simulink model "harmonics"  (R2025b)
settings: Solver=ode14x  StartTime=0.0  StopTime=0.2  FixedStep=1e-5  RelTol=1e-3
values from neighbouring files (symbols this model uses):
  f = 50.0    [ctrlSys.sldd]
  Ts_local = 1.0E-5    [ctrlSys.sldd]
libraries: eeRmsMeasurement x2
settings Model: DataDictionary=ctrlSys.sldd  Creator=LYG  LastModifiedBy=i336

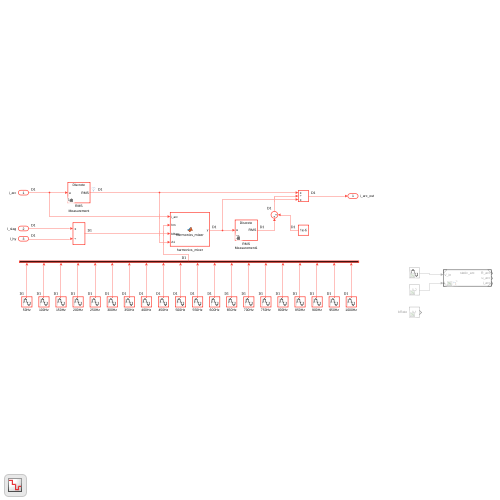
[thumbnail: Simulink's stored preview of the top-level diagram]
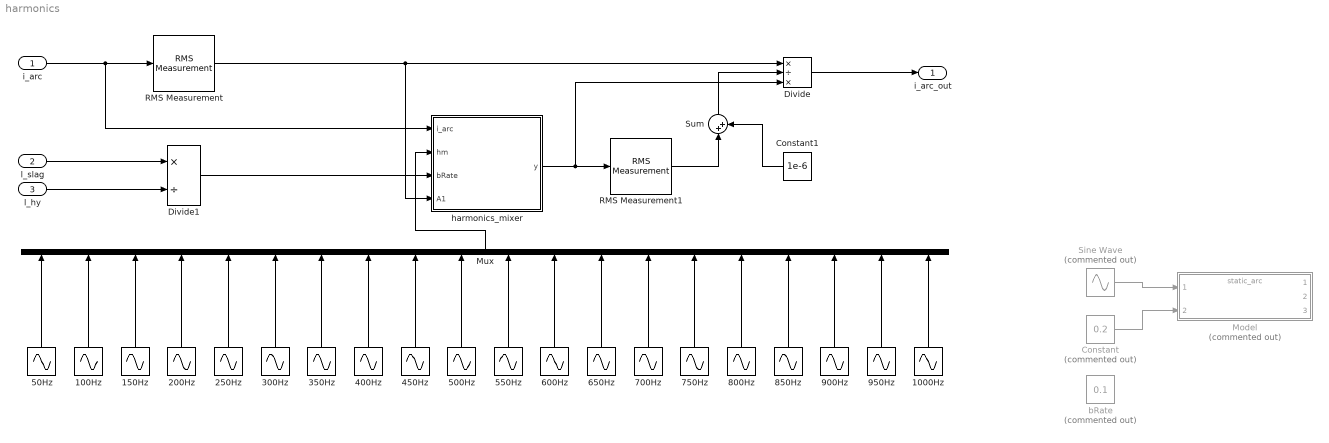
== system harmonics ==
  i_arc : Inport
  l_slag : Inport  Port=2
  l_hy : Inport  Port=3  PortDimensions=3
  1000Hz : Sin  Frequency=2 * pi * f * 20  Phase=-0.6225  SampleTime=Ts_local
  100Hz : Sin  Frequency=2 * pi * f * 2  Phase=-0.4679  SampleTime=Ts_local
  150Hz : Sin  Frequency=2 * pi * f * 3  Phase=-0.8069  SampleTime=Ts_local
  200Hz : Sin  Frequency=2 * pi * f * 4  Phase=0.0685  SampleTime=Ts_local
  250Hz : Sin  Frequency=2 * pi * f * 5  Phase=-1.3175  SampleTime=Ts_local
  300Hz : Sin  Frequency=2 * pi * f * 6  Phase=-0.0827  SampleTime=Ts_local
  350Hz : Sin  Frequency=2 * pi * f * 7  Phase=-1.1120  SampleTime=Ts_local
  400Hz : Sin  Frequency=2 * pi * f * 8  Phase=-0.4285  SampleTime=Ts_local
  450Hz : Sin  Frequency=2 * pi * f * 9  Phase=-1.5794  SampleTime=Ts_local
  500Hz : Sin  Frequency=2 * pi * f * 10  Phase=-0.2913  SampleTime=Ts_local
  50Hz : Sin  Frequency=2 * pi * f * 1  Phase=-2.2678  SampleTime=Ts_local
  550Hz : Sin  Frequency=2 * pi * f * 11  Phase=-1.9727  SampleTime=Ts_local
  600Hz : Sin  Frequency=2 * pi * f * 12  Phase=-0.4659  SampleTime=Ts_local
  650Hz : Sin  Frequency=2 * pi * f * 13  Phase=-2.1009  SampleTime=Ts_local
  700Hz : Sin  Frequency=2 * pi * f * 14  Phase=-0.5103  SampleTime=Ts_local
  750Hz : Sin  Frequency=2 * pi * f * 15  Phase=-2.4781  SampleTime=Ts_local
  800Hz : Sin  Frequency=2 * pi * f * 16  Phase=-0.5504  SampleTime=Ts_local
  850Hz : Sin  Frequency=2 * pi * f * 17  Phase=-2.8439  SampleTime=Ts_local
  900Hz : Sin  Frequency=2 * pi * f * 18  Phase=-0.6115  SampleTime=Ts_local
  950Hz : Sin  Frequency=2 * pi * f * 19  Phase=3.1081  SampleTime=Ts_local
  Constant : Constant  Commented=on  Value=0.2  SampleTime=1e-5
  Constant1 : Constant  Value=1e-6  SampleTime=Ts_local
  Divide : Product  Inputs=*/*
  Divide1 : Product  Inputs=*/
  Model : ModelReference  Commented=on  ModelNameDialog=static_arc.slx  SimulationMode=Normal  ModelReferenceVersion=1.10
  Mux : Mux  Inputs=20
  RMS Measurement : eeRmsMeasurement/RMS Measurement  LabelModeActiveChoice=Total  F=f  SpecifyHarmonics=off  K=[0 1 2]  Ts=Ts_local
      settings: LibrarySourceBlock=|
      | ee_sl_lib/Measurements/RMS
      | Measurement
  RMS Measurement1 : eeRmsMeasurement/RMS Measurement  LabelModeActiveChoice=Total  F=f  SpecifyHarmonics=off  K=[0 1]  Ts=Ts_local
      settings: LibrarySourceBlock=|
      | ee_sl_lib/Measurements/RMS
      | Measurement
  Sine Wave : Sin  Commented=on  Amplitude=sqrt(2) * 650  Frequency=2 * pi * 50  SampleTime=1e-5
  Sum : Sum  Inputs=|++
  bRate : Constant  Commented=on  Value=0.1  SampleTime=1e-5
  harmonics_mixer : MATLAB Function  TreatAsAtomicUnit=on  SystemSampleTime=Ts_local
  i_arc_out : Outport
  wires:
  Sine Wave/1 -> Model/1
  Constant/1 -> Model/2
  50Hz/1 -> Mux/1
  100Hz/1 -> Mux/2
  150Hz/1 -> Mux/3
  200Hz/1 -> Mux/4
  250Hz/1 -> Mux/5
  300Hz/1 -> Mux/6
  350Hz/1 -> Mux/7
  400Hz/1 -> Mux/8
  450Hz/1 -> Mux/9
  500Hz/1 -> Mux/10
  Mux/1 -> harmonics_mixer/2(hm)
  RMS Measurement/1 -> Divide/1, harmonics_mixer/4(A1)
  harmonics_mixer/1(y) -> Divide/3, RMS Measurement1/1
  Sum/1 -> Divide/2
  RMS Measurement1/1 -> Sum/1
  Constant1/1 -> Sum/2
  550Hz/1 -> Mux/11
  600Hz/1 -> Mux/12
  650Hz/1 -> Mux/13
  700Hz/1 -> Mux/14
  750Hz/1 -> Mux/15
  800Hz/1 -> Mux/16
  850Hz/1 -> Mux/17
  900Hz/1 -> Mux/18
  1000Hz/1 -> Mux/20
  950Hz/1 -> Mux/19
  i_arc/1 -> harmonics_mixer/1(i_arc), RMS Measurement/1
  l_slag/1 -> Divide1/1
  Divide1/1 -> harmonics_mixer/3(bRate)
  l_hy/1 -> Divide1/2
  Divide/1 -> i_arc_out/1

== matlab function harmonics/harmonics_mixer ==
  data: i_arc input size=[3 1]; hm input; y output; bRate input size=[3 1]; A1 input size=[3 1]
function y = harmonics_mixer(i_arc, hm, bRate, A1)
    i_arc = i_arc(:);
    hm = hm(:);
    bRate = bRate(:);
    A1 = A1(:);

    N = 20; % Number of harmonics to add
    alpha = 0.5 + 5 * bRate; % Decay factor for the harmonics
    c = 1e4 * (1 - bRate);

    Ahm_ls = zeros(3, N);
    for i = 1 : N
        if mod(i, 2) == 0
            Ahm_ls(:, i) = A1 .* exp(-alpha * (i - 1)) + c;
        else
            Ahm_ls(:, i) = c;
        end
    end

    Ah = zeros(3, 1);
    for i = 1:length(hm)
        Ah = Ah + hm(i) * Ahm_ls(:, i);
    end

    y = Ah + i_arc;
end
